simulink model "Counter_up"  (R2016b)
settings: Solver=VariableStepAuto  StartTime=0.0  StopTime=10.0  RelTol=1e-3
settings Model: Creator=Saher Ghanem  LastModifiedBy=Saher Ghanem

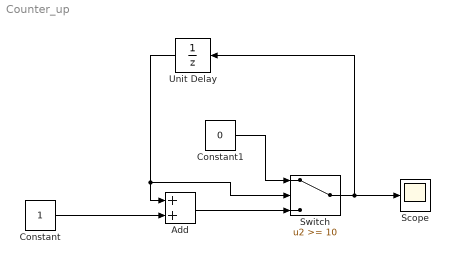
== system Counter_up ==
  Add : Sum
  Constant : Constant
  Constant1 : Constant  Value=0
  Scope : Scope
  Switch : Switch  Threshold=10
  Unit Delay : UnitDelay  SampleTime=-1
  wires:
  Constant/1 -> Add/2
  Unit Delay/1 -> Switch/2, Add/1
  Constant1/1 -> Switch/1
  Add/1 -> Switch/3
  Switch/1 -> Scope/1, Unit Delay/1
